simulink model "wieght_functions"  (R2021b)
settings: Solver=VariableStepAuto  StartTime=0.0  StopTime=10.0  RelTol=1e-3
settings Model: Creator=vkad  LastModifiedBy=vkad

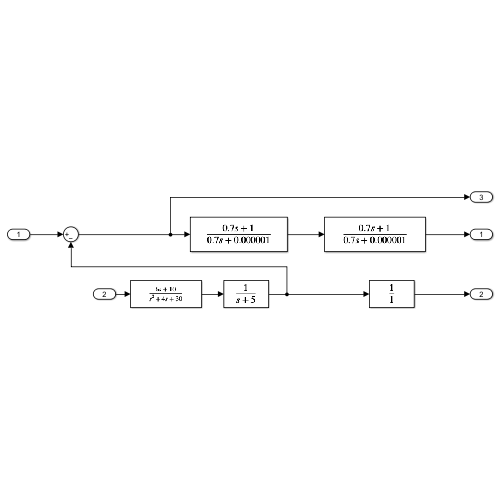
[thumbnail: Simulink's stored preview of the top-level diagram]
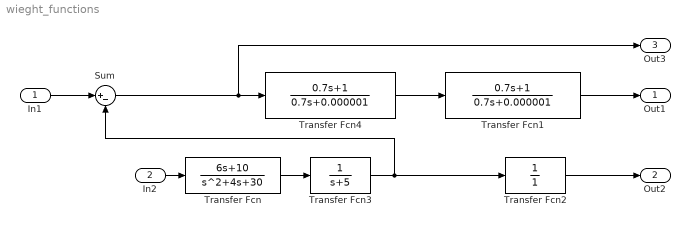
== system wieght_functions ==
  In1 : Inport
  In2 : Inport  Port=2
  Sum : Sum  Inputs=|+-
  Transfer Fcn : TransferFcn  Numerator=[6 10]  Denominator=[1 4 30]
  Transfer Fcn1 : TransferFcn  Numerator=[0.7 1]  Denominator=[0.7 0.000001]
  Transfer Fcn2 : TransferFcn  Denominator=[1]
  Transfer Fcn3 : TransferFcn  Denominator=[1 5]
  Transfer Fcn4 : TransferFcn  Numerator=[0.7 1]  Denominator=[0.7 0.000001]
  Out1 : Outport
  Out2 : Outport  Port=2
  Out3 : Outport  Port=3
  wires:
  Transfer Fcn/1 -> Transfer Fcn3/1
  In1/1 -> Sum/1
  In2/1 -> Transfer Fcn/1
  Transfer Fcn3/1 -> Transfer Fcn2/1, Sum/2
  Transfer Fcn1/1 -> Out1/1
  Sum/1 -> Transfer Fcn4/1, Out3/1
  Transfer Fcn2/1 -> Out2/1
  Transfer Fcn4/1 -> Transfer Fcn1/1
